simulink model "PMSM_Optimization"  (R2024a)
settings: Solver=VariableStepAuto  StartTime=0.0  StopTime=2  RelTol=1e-3
undefined symbols (not defined in the file): a, b, Kd, Ki, Kp
libraries: checkpacklib x4, fod x1, slpidlib x1
settings Model: Creator=CadenceHB04  LastModifiedBy=CadenceHB04

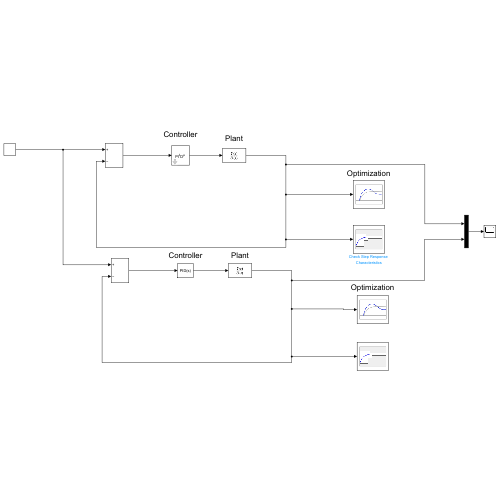
[thumbnail: Simulink's stored preview of the top-level diagram]
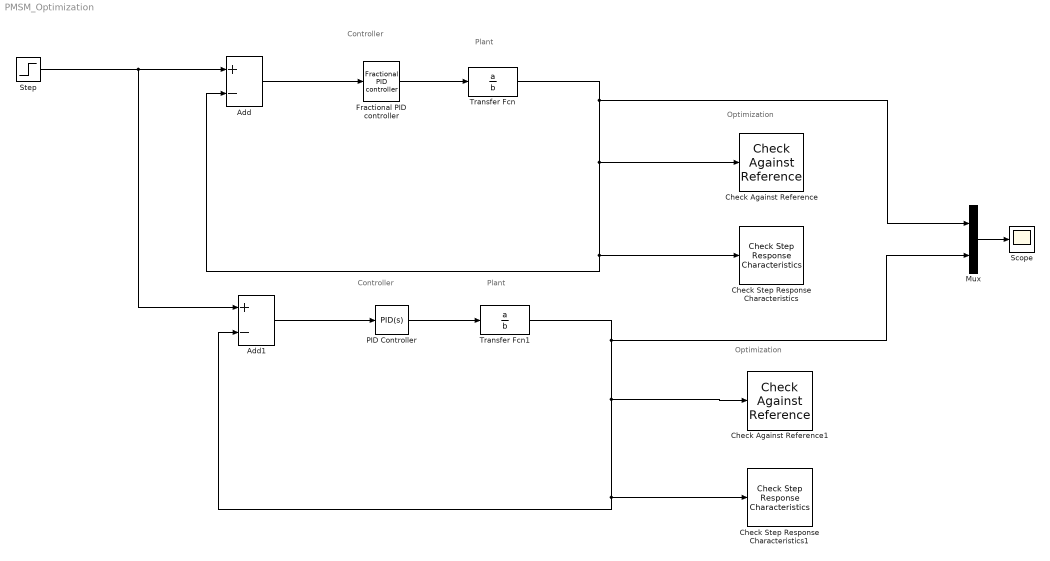
== system PMSM_Optimization ==
  note: Optimization
  note: Plant
  note: Plant
  note: Controller
  note: Controller
  note: Optimization
  Add : Sum  Inputs=+-
  Add1 : Sum  Inputs=+-
  Check Against Reference : checkpacklib/Check Against Reference  InstantiateOnLoad=on  enabled=on  stopWhenAssertionFail=off  export=off  ViewDlgPos=[]  OpenViewOnLoad=off  LaunchViewOnOpen=off  TimeUnits=seconds  EnableReferenceBound=on  AbsTolerance=eps^(1/3)  RelTolerance=0.01  ReferenceTimes=linspace(0,10)  ReferenceAmplitudes=1-exp(-linspace(0,10)/2)
      settings: LibrarySourceBlock=sdolib/Signal Constraints/Check Against Reference
  Check Against Reference1 : checkpacklib/Check Against Reference  InstantiateOnLoad=on  enabled=on  stopWhenAssertionFail=off  export=off  ViewDlgPos=[]  OpenViewOnLoad=off  LaunchViewOnOpen=off  TimeUnits=seconds  EnableReferenceBound=on  AbsTolerance=eps^(1/3)  RelTolerance=0.01  ReferenceTimes=linspace(0,10)  ReferenceAmplitudes=1-exp(-linspace(0,10)/2)
      settings: LibrarySourceBlock=sdolib/Signal Constraints/Check Against Reference
  Check Step Response Characteristics : checkpacklib/Check Step Response  Characteristics  InstantiateOnLoad=on  enabled=on  stopWhenAssertionFail=off  export=off  ViewDlgPos=[]  OpenViewOnLoad=off  LaunchViewOnOpen=off  TimeUnits=seconds  EnableStepResponseBound=on  InitialValue=0  FinalValue=1  StepTime=0  RiseTime=0.00001  PercentRise=80  SettlingTime=0.00002  PercentSettling=1  PercentOvershoot=1  PercentUndershoot=1
      settings: LibrarySourceBlock=|
      | sdolib/Signal Constraints/Check Step Response
      | Characteristics
  Check Step Response Characteristics1 : checkpacklib/Check Step Response  Characteristics  InstantiateOnLoad=on  enabled=on  stopWhenAssertionFail=off  export=off  ViewDlgPos=[]  OpenViewOnLoad=off  LaunchViewOnOpen=off  TimeUnits=seconds  EnableStepResponseBound=on  InitialValue=0  FinalValue=1  StepTime=0  RiseTime=0.00001  PercentRise=80  SettlingTime=0.00002  PercentSettling=1  PercentOvershoot=1  PercentUndershoot=1
      settings: LibrarySourceBlock=|
      | sdolib/Signal Constraints/Check Step Response
      | Characteristics
  Fractional PID controller : fod/Fractional PID controller  Kp=Kp  Ki=Ki  lambda=lamda  Kd=Kd  mic=mu  freqRange=[0.001, 1000]  N=5
      settings: SourceProductName=FOMCON Toolbox
  Mux : Mux  Inputs=2
  PID Controller : slpidlib/PID Controller  Controller=PID  Form=Parallel  TimeDomain=Continuous-time  UseExternalTs=off  SampleTime=-1  IntegratorMethod=Forward Euler  FilterMethod=Forward Euler  ControllerParametersSource=internal  P=1  I=1  UseKiTs=off  D=0  UseExternalDerivativeSource=off  N=100  UseFilter=on  TunerSelectOption=Transfer Function Based (PID Tuner App)  InitialConditionSource=internal  InitialConditionForIntegrator=0  InitialConditionForFilter=0  DifferentiatorICPrevScaledInput=0  ExternalReset=none  TrackingMode=off  Kt=1  LimitOutput=off  SatLimitsSource=internal  UpperSaturationLimit=inf  LowerSaturationLimit=-inf  LinearizeAsGain=on  AntiWindupMode=none  Kb=1  LimitIntegrator=off  UpperIntegratorSaturationLimit=inf  LowerIntegratorSaturationLimit=-inf  POutMin=[]  POutMax=[]  IOutMin=[]  IOutMax=[]  DOutMin=[]  DOutMax=[]  NOutMin=[]  NOutMax=[]  SumOutMin=[]  SumOutMax=[]  SaturationOutMin=[]  SaturationOutMax=[]  PParamMin=[]  PParamMax=[]  IParamMin=[]  IParamMax=[]  DParamMin=[]  DParamMax=[]  NParamMin=[]  NParamMax=[]  KbParamMin=[]  KbParamMax=[]  KtParamMin=[]  KtParamMax=[]  KbOutMin=[]  KbOutMax=[]  KtOutMin=[]  KtOutMax=[]  IntegratorOutMin=[]  IntegratorOutMax=[]  FilterOutMin=[]  FilterOutMax=[]  SumI1OutMin=[]  SumI1OutMax=[]  SumI2OutMin=[]  SumI2OutMax=[]  SumI3OutMin=[]  SumI3OutMax=[]  SumI4OutMin=[]  SumI4OutMax=[]  SumDOutMin=[]  SumDOutMax=[]  DifferentiatorOutMin=[]  DifferentiatorOutMax=[]  FilterDiffOutCoefMin=[]  FilterDiffOutCoefMax=[]  ReciprocalOutMin=[]  ReciprocalOutMax=[]  SumDenOutMin=[]  SumDenOutMax=[]  SumNumOutMin=[]  SumNumOutMax=[]  DivideOutMin=[]  DivideOutMax=[]  UdiffTsProdOutMin=[]  UdiffTsProdOutMax=[]  NTsProdOutMin=[]  NTsProdOutMax=[]  UintegralTsProdOutMin=[]  UintegralTsProdOutMax=[]  UngainTsProdOutMin=[]  UngainTsProdOutMax=[]  ClampingZeroOutDataTypeStr=Inherit: Inherit via back propagation  ClampingZeroOutMin=[]  ClampingZeroOutMax=[]  FilterDenConstantOutDataTypeStr=Inherit: Inherit via back propagation  FilterDenConstantOutMin=[]  FilterDenConstantOutMax=[]  PCopyOutDataTypeStr=Inherit: Inherit via back propagation  PCopyOutMin=[]  PCopyOutMax=[]  NCopyOutDataTypeStr=Inherit: Inherit via back propagation  NCopyOutMin=[]  NCopyOutMax=[]  IntegratorContinuousStateAttributes=''  IntegratorStateMustResolveToSignalObject=off  IntegratorRTWStateStorageClass=Auto  FilterContinuousStateAttributes=''  FilterStateMustResolveToSignalObject=off  FilterRTWStateStorageClass=Auto  ParallelPVariant=InternalParameters  IdealPVariant=Disabled  IVariant=InternalParameters  DVariant=InternalParameters  IntegratorVariant=Continuous  SatVariant=Disabled  AWVariant=Passthrough  PCopyVariant=Disabled  TRVariant=Disabled  FdbkBlocksVariant=Forward  IdealPFdbkVariant=Disabled  SatFdbkVariant=Disabled  DerivativeFilterVariant=ContFilter  NVariant=InternalParameters  NCopyVariant=Disabled  FilterICVariant=InternalICsFilter  IntegratorICVariant=InternalICs  ExternalResetVariant=Disabled  TRSumVariant=Passthrough  SumFdbkVariant=Disabled  SumVariant=Sum_PID  TsampFilterVariant=InternalTs  TsampNgainVariant=Passthrough  TsampIntegralVariant=Passthrough  ExternalSaturationOutDataTypeStr=Inherit: Same as second input  DerivativeSourceVariant=ErrorSignal
  Scope : Scope
  Step : Step  Time=10  Before=1  SampleTime=0
  Transfer Fcn : TransferFcn  Numerator=a  Denominator=b
  Transfer Fcn1 : TransferFcn  Numerator=a  Denominator=b
  wires:
  Step/1 -> Add/1, Add1/1
  Transfer Fcn/1 -> Add/2, Check Step Response Characteristics/1, Check Against Reference/1, Mux/1
  Fractional PID controller/1 -> Transfer Fcn/1
  Add/1 -> Fractional PID controller/1
  PID Controller/1 -> Transfer Fcn1/1
  Add1/1 -> PID Controller/1
  Transfer Fcn1/1 -> Mux/2, Check Against Reference1/1, Check Step Response Characteristics1/1, Add1/2
  Mux/1 -> Scope/1
